simulink model "BrkPed_SetData"  (R2016b)
settings: configuration reference "CodeGenConfigSet" (kept outside this file)
settings Model: Creator=lenovo  LastModifiedBy=lenovo
settings ConfigSetRef: SourceLocation=Base Workspace

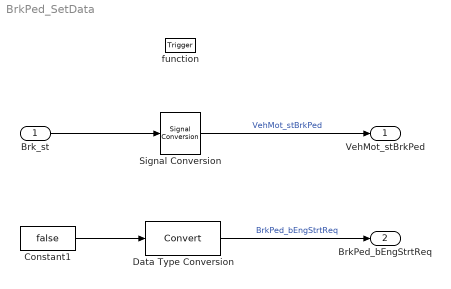
== system BrkPed_SetData ==
  Brk_st : Inport  Description=Brake switch state  OutMin=0  OutMax=255  OutDataTypeStr=State_uint8
  function : TriggerPort  TriggerType=function-call  VariantControl=Variant
  Constant1 : Constant  RequirementInfo={'other' 'APP_requirements.doc' '@Simulink_requirement_item_25' 'true' '手动开关' '' } %GIDa_27444533_52c7_4a80_b10c_6ba2f02406f2  Value=false  OutDataTypeStr=Inherit: Inherit via back propagation
  Data Type Conversion : DataTypeConversion
  Signal Conversion : SignalConversion  OverrideOpt=off
  VehMot_stBrkPed : Outport  Description=Information brake pedal pressed  OutMin=0  OutMax=255  OutDataTypeStr=State_uint8
  BrkPed_bEngStrtReq : Outport  Description=Start request brake system  Port=2  OutMin=0  OutMax=1  OutDataTypeStr=boolean
  wires:
  Signal Conversion/1 -> VehMot_stBrkPed/1  "VehMot_stBrkPed"
  Constant1/1 -> Data Type Conversion/1
  Brk_st/1 -> Signal Conversion/1
  Data Type Conversion/1 -> BrkPed_bEngStrtReq/1  "BrkPed_bEngStrtReq"
